simulink model "plant"  (R2016b)
settings: Solver=VariableStepAuto  StartTime=0.0  StopTime=10.0  RelTol=1e-3
values from neighbouring files (symbols this model uses):
  Ts = 0.04    [LPV_Torsional.m]    (also in main.m = G1.Ts)
libraries: simulink x1
settings Model: Creator=akarimi  LastModifiedBy=akarimi

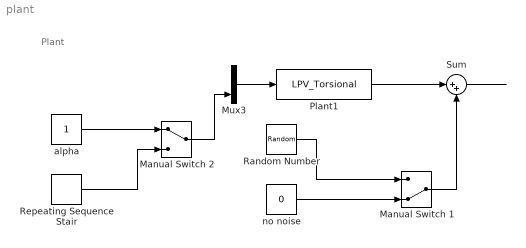
== system plant ==
  note: Plant
  Manual Switch 1 : ManualSwitch  CurrentSetting=0
  Manual Switch 2 : ManualSwitch
  Mux3 : Mux  Inputs=2
  Plant1 : S-Function  FunctionName=LPV_Torsional  SFunctionDeploymentMode=off  EnableBusSupport=off
  Random Number : RandomNumber  Variance=0.00001  SampleTime=Ts
  Repeating Sequence Stair : simulink/Sources/Repeating Sequence Stair  OutValues=[-1 1 0.5 -0.5 1 0].'  tsamp=25  OutMin=[]  OutMax=[]  OutDataTypeStr=double  OutputDataTypeScalingMode=double  OutDataType=fixdt(0,8)  ConRadixGroup=Best Precision: Vector-wise  OutScaling=2^-12
  Sum : Sum  Inputs=|++
  alpha : Constant
  "no noise " : Constant  Value=0
  wires:
  alpha/1 -> Manual Switch 2/1
  Repeating Sequence Stair/1 -> Manual Switch 2/2
  Random Number/1 -> Manual Switch 1/1
  Manual Switch 1/1 -> Sum/2
  "no noise "/1 -> Manual Switch 1/2
  Manual Switch 2/1 -> Mux3/2
  ? -> Mux3/1
  Plant1/1 -> Sum/1
  Mux3/1 -> Plant1/1
  Sum/1 -> ?
